simulink library "xblocks_library_pfbs"  (Simulink 7.6)
settings: Solver=ode45  SolverMode=SingleTasking  StartTime=0.0  StopTime=10.0  RelTol=1e-3
libraries: xbsIndex_r4 x369, monroe_library x47
(part 7 of 7)

== system xblocks_library_pfbs/pfb_fir/pfb_row_22/tap_split_2 ==
  inport : Inport
  Reinterp1 : xbsIndex_r4/Reinterpret  force_arith_type=on  arith_type="Signed  (2's comp)"  force_bin_pt=on  bin_pt=7  block_type=reinterpret
  Reinterp2 : xbsIndex_r4/Reinterpret  force_arith_type=on  arith_type="Signed  (2's comp)"  force_bin_pt=on  bin_pt=7  block_type=reinterpret
  Slice1 : xbsIndex_r4/Slice  nbits=8  boolean_output=off  mode=Upper Bit Location + Width  bit1=-0  base1=MSB of Input  bit0=0  base0=LSB of Input  dbl_ovrd=off  block_type=slice
  Slice2 : xbsIndex_r4/Slice  nbits=8  boolean_output=off  mode=Upper Bit Location + Width  bit1=-8  base1=MSB of Input  bit0=0  base0=LSB of Input  dbl_ovrd=off  block_type=slice
  outport1 : Outport
  outport2 : Outport  Port=2
  wires:
  inport/1 -> Slice2/1, Slice1/1
  Reinterp2/1 -> outport2/1
  Slice2/1 -> Reinterp2/1  "slice_out2"
  Reinterp1/1 -> outport1/1
  Slice1/1 -> Reinterp1/1  "slice_out1"

== system xblocks_library_pfbs/pfb_fir_real/coeff_gen_0_7/cram_lower ==
  in0 : Inport
  in1 : Inport  Port=2
  in2 : Inport  Port=3
  in3 : Inport  Port=4
  concat : xbsIndex_r4/Concat  num_inputs=4  dbl_ovrd=off  block_type=concat
  reinterpret_{1..4} (4 alike) : xbsIndex_r4/Reinterpret  force_arith_type=on  arith_type=Unsigned  force_bin_pt=on  bin_pt=0  block_type=reinterpret
  out : Outport
  wires:
  concat/1 -> out/1
  reinterpret_4/1 -> concat/4
  reinterpret_3/1 -> concat/3
  reinterpret_2/1 -> concat/2
  reinterpret_1/1 -> concat/1
  in3/1 -> reinterpret_4/1
  in2/1 -> reinterpret_3/1
  in1/1 -> reinterpret_2/1
  in0/1 -> reinterpret_1/1

== system xblocks_library_pfbs/pfb_fir_real/coeff_gen_0_7/cram_upper ==
  in0 : Inport
  in1 : Inport  Port=2
  in2 : Inport  Port=3
  in3 : Inport  Port=4
  concat : xbsIndex_r4/Concat  num_inputs=4  dbl_ovrd=off  block_type=concat
  reinterpret_{1..4} (4 alike) : xbsIndex_r4/Reinterpret  force_arith_type=on  arith_type=Unsigned  force_bin_pt=on  bin_pt=0  block_type=reinterpret
  out : Outport
  wires:
  concat/1 -> out/1
  reinterpret_4/1 -> concat/4
  reinterpret_3/1 -> concat/3
  reinterpret_2/1 -> concat/2
  reinterpret_1/1 -> concat/1
  in3/1 -> reinterpret_4/1
  in2/1 -> reinterpret_3/1
  in1/1 -> reinterpret_2/1
  in0/1 -> reinterpret_1/1

== system xblocks_library_pfbs/pfb_fir_real/coeff_gen_1_6/cram_lower ==
  in0 : Inport
  in1 : Inport  Port=2
  in2 : Inport  Port=3
  in3 : Inport  Port=4
  concat : xbsIndex_r4/Concat  num_inputs=4  dbl_ovrd=off  block_type=concat
  reinterpret_{1..4} (4 alike) : xbsIndex_r4/Reinterpret  force_arith_type=on  arith_type=Unsigned  force_bin_pt=on  bin_pt=0  block_type=reinterpret
  out : Outport
  wires:
  concat/1 -> out/1
  reinterpret_4/1 -> concat/4
  reinterpret_3/1 -> concat/3
  reinterpret_2/1 -> concat/2
  reinterpret_1/1 -> concat/1
  in3/1 -> reinterpret_4/1
  in2/1 -> reinterpret_3/1
  in1/1 -> reinterpret_2/1
  in0/1 -> reinterpret_1/1

== system xblocks_library_pfbs/pfb_fir_real/coeff_gen_1_6/cram_upper ==
  in0 : Inport
  in1 : Inport  Port=2
  in2 : Inport  Port=3
  in3 : Inport  Port=4
  concat : xbsIndex_r4/Concat  num_inputs=4  dbl_ovrd=off  block_type=concat
  reinterpret_{1..4} (4 alike) : xbsIndex_r4/Reinterpret  force_arith_type=on  arith_type=Unsigned  force_bin_pt=on  bin_pt=0  block_type=reinterpret
  out : Outport
  wires:
  concat/1 -> out/1
  reinterpret_4/1 -> concat/4
  reinterpret_3/1 -> concat/3
  reinterpret_2/1 -> concat/2
  reinterpret_1/1 -> concat/1
  in3/1 -> reinterpret_4/1
  in2/1 -> reinterpret_3/1
  in1/1 -> reinterpret_2/1
  in0/1 -> reinterpret_1/1

== system xblocks_library_pfbs/pfb_fir_real/coeff_gen_2_5/cram_lower ==
  in0 : Inport
  in1 : Inport  Port=2
  in2 : Inport  Port=3
  in3 : Inport  Port=4
  concat : xbsIndex_r4/Concat  num_inputs=4  dbl_ovrd=off  block_type=concat
  reinterpret_{1..4} (4 alike) : xbsIndex_r4/Reinterpret  force_arith_type=on  arith_type=Unsigned  force_bin_pt=on  bin_pt=0  block_type=reinterpret
  out : Outport
  wires:
  concat/1 -> out/1
  reinterpret_4/1 -> concat/4
  reinterpret_3/1 -> concat/3
  reinterpret_2/1 -> concat/2
  reinterpret_1/1 -> concat/1
  in3/1 -> reinterpret_4/1
  in2/1 -> reinterpret_3/1
  in1/1 -> reinterpret_2/1
  in0/1 -> reinterpret_1/1

== system xblocks_library_pfbs/pfb_fir_real/coeff_gen_2_5/cram_upper ==
  in0 : Inport
  in1 : Inport  Port=2
  in2 : Inport  Port=3
  in3 : Inport  Port=4
  concat : xbsIndex_r4/Concat  num_inputs=4  dbl_ovrd=off  block_type=concat
  reinterpret_{1..4} (4 alike) : xbsIndex_r4/Reinterpret  force_arith_type=on  arith_type=Unsigned  force_bin_pt=on  bin_pt=0  block_type=reinterpret
  out : Outport
  wires:
  concat/1 -> out/1
  reinterpret_4/1 -> concat/4
  reinterpret_3/1 -> concat/3
  reinterpret_2/1 -> concat/2
  reinterpret_1/1 -> concat/1
  in3/1 -> reinterpret_4/1
  in2/1 -> reinterpret_3/1
  in1/1 -> reinterpret_2/1
  in0/1 -> reinterpret_1/1

== system xblocks_library_pfbs/pfb_fir_real/coeff_gen_3_4/cram_lower ==
  in0 : Inport
  in1 : Inport  Port=2
  in2 : Inport  Port=3
  in3 : Inport  Port=4
  concat : xbsIndex_r4/Concat  num_inputs=4  dbl_ovrd=off  block_type=concat
  reinterpret_{1..4} (4 alike) : xbsIndex_r4/Reinterpret  force_arith_type=on  arith_type=Unsigned  force_bin_pt=on  bin_pt=0  block_type=reinterpret
  out : Outport
  wires:
  concat/1 -> out/1
  reinterpret_4/1 -> concat/4
  reinterpret_3/1 -> concat/3
  reinterpret_2/1 -> concat/2
  reinterpret_1/1 -> concat/1
  in3/1 -> reinterpret_4/1
  in2/1 -> reinterpret_3/1
  in1/1 -> reinterpret_2/1
  in0/1 -> reinterpret_1/1

== system xblocks_library_pfbs/pfb_fir_real/coeff_gen_3_4/cram_upper ==
  in0 : Inport
  in1 : Inport  Port=2
  in2 : Inport  Port=3
  in3 : Inport  Port=4
  concat : xbsIndex_r4/Concat  num_inputs=4  dbl_ovrd=off  block_type=concat
  reinterpret_{1..4} (4 alike) : xbsIndex_r4/Reinterpret  force_arith_type=on  arith_type=Unsigned  force_bin_pt=on  bin_pt=0  block_type=reinterpret
  out : Outport
  wires:
  concat/1 -> out/1
  reinterpret_4/1 -> concat/4
  reinterpret_3/1 -> concat/3
  reinterpret_2/1 -> concat/2
  reinterpret_1/1 -> concat/1
  in3/1 -> reinterpret_4/1
  in2/1 -> reinterpret_3/1
  in1/1 -> reinterpret_2/1
  in0/1 -> reinterpret_1/1

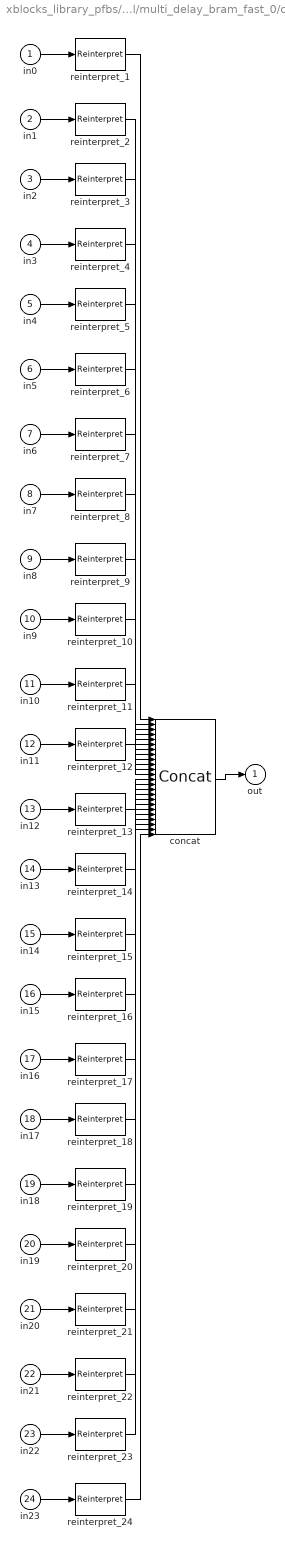
== system xblocks_library_pfbs/pfb_fir_real/multi_delay_bram_fast_0/cram ==
  in0 : Inport
  in1 : Inport  Port=2
  in2 : Inport  Port=3
  in3 : Inport  Port=4
  in4 : Inport  Port=5
  in5 : Inport  Port=6
  in6 : Inport  Port=7
  in7 : Inport  Port=8
  in8 : Inport  Port=9
  in9 : Inport  Port=10
  in10 : Inport  Port=11
  in11 : Inport  Port=12
  in12 : Inport  Port=13
  in13 : Inport  Port=14
  in14 : Inport  Port=15
  in15 : Inport  Port=16
  in16 : Inport  Port=17
  in17 : Inport  Port=18
  in18 : Inport  Port=19
  in19 : Inport  Port=20
  in20 : Inport  Port=21
  in21 : Inport  Port=22
  in22 : Inport  Port=23
  in23 : Inport  Port=24
  concat : xbsIndex_r4/Concat  num_inputs=24  dbl_ovrd=off  block_type=concat
  reinterpret_{1..24} (24 alike) : xbsIndex_r4/Reinterpret  force_arith_type=on  arith_type=Unsigned  force_bin_pt=on  bin_pt=0  block_type=reinterpret
  out : Outport
  wires:
  concat/1 -> out/1
  reinterpret_24/1 -> concat/24
  reinterpret_23/1 -> concat/23
  reinterpret_22/1 -> concat/22
  reinterpret_21/1 -> concat/21
  reinterpret_20/1 -> concat/20
  reinterpret_19/1 -> concat/19
  reinterpret_18/1 -> concat/18
  reinterpret_17/1 -> concat/17
  reinterpret_16/1 -> concat/16
  reinterpret_15/1 -> concat/15
  reinterpret_14/1 -> concat/14
  reinterpret_13/1 -> concat/13
  reinterpret_12/1 -> concat/12
  reinterpret_11/1 -> concat/11
  reinterpret_10/1 -> concat/10
  reinterpret_9/1 -> concat/9
  reinterpret_8/1 -> concat/8
  reinterpret_7/1 -> concat/7
  reinterpret_6/1 -> concat/6
  reinterpret_5/1 -> concat/5
  reinterpret_4/1 -> concat/4
  reinterpret_3/1 -> concat/3
  reinterpret_2/1 -> concat/2
  reinterpret_1/1 -> concat/1
  in23/1 -> reinterpret_24/1
  in22/1 -> reinterpret_23/1
  in21/1 -> reinterpret_22/1
  in20/1 -> reinterpret_21/1
  in19/1 -> reinterpret_20/1
  in18/1 -> reinterpret_19/1
  in17/1 -> reinterpret_18/1
  in16/1 -> reinterpret_17/1
  in15/1 -> reinterpret_16/1
  in14/1 -> reinterpret_15/1
  in13/1 -> reinterpret_14/1
  in12/1 -> reinterpret_13/1
  in11/1 -> reinterpret_12/1
  in10/1 -> reinterpret_11/1
  in9/1 -> reinterpret_10/1
  in8/1 -> reinterpret_9/1
  in7/1 -> reinterpret_8/1
  in6/1 -> reinterpret_7/1
  in5/1 -> reinterpret_6/1
  in4/1 -> reinterpret_5/1
  in3/1 -> reinterpret_4/1
  in2/1 -> reinterpret_3/1
  in1/1 -> reinterpret_2/1
  in0/1 -> reinterpret_1/1

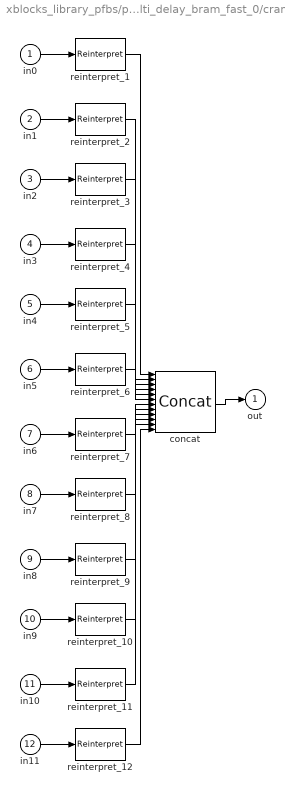
== system xblocks_library_pfbs/pfb_fir_real/multi_delay_bram_fast_0/cram_all ==
  in0 : Inport
  in1 : Inport  Port=2
  in2 : Inport  Port=3
  in3 : Inport  Port=4
  in4 : Inport  Port=5
  in5 : Inport  Port=6
  in6 : Inport  Port=7
  in7 : Inport  Port=8
  in8 : Inport  Port=9
  in9 : Inport  Port=10
  in10 : Inport  Port=11
  in11 : Inport  Port=12
  concat : xbsIndex_r4/Concat  num_inputs=12  dbl_ovrd=off  block_type=concat
  reinterpret_{1..12} (12 alike) : xbsIndex_r4/Reinterpret  force_arith_type=on  arith_type=Unsigned  force_bin_pt=on  bin_pt=0  block_type=reinterpret
  out : Outport
  wires:
  concat/1 -> out/1
  reinterpret_12/1 -> concat/12
  reinterpret_11/1 -> concat/11
  reinterpret_10/1 -> concat/10
  reinterpret_9/1 -> concat/9
  reinterpret_8/1 -> concat/8
  reinterpret_7/1 -> concat/7
  reinterpret_6/1 -> concat/6
  reinterpret_5/1 -> concat/5
  reinterpret_4/1 -> concat/4
  reinterpret_3/1 -> concat/3
  reinterpret_2/1 -> concat/2
  reinterpret_1/1 -> concat/1
  in11/1 -> reinterpret_12/1
  in10/1 -> reinterpret_11/1
  in9/1 -> reinterpret_10/1
  in8/1 -> reinterpret_9/1
  in7/1 -> reinterpret_8/1
  in6/1 -> reinterpret_7/1
  in5/1 -> reinterpret_6/1
  in4/1 -> reinterpret_5/1
  in3/1 -> reinterpret_4/1
  in2/1 -> reinterpret_3/1
  in1/1 -> reinterpret_2/1
  in0/1 -> reinterpret_1/1

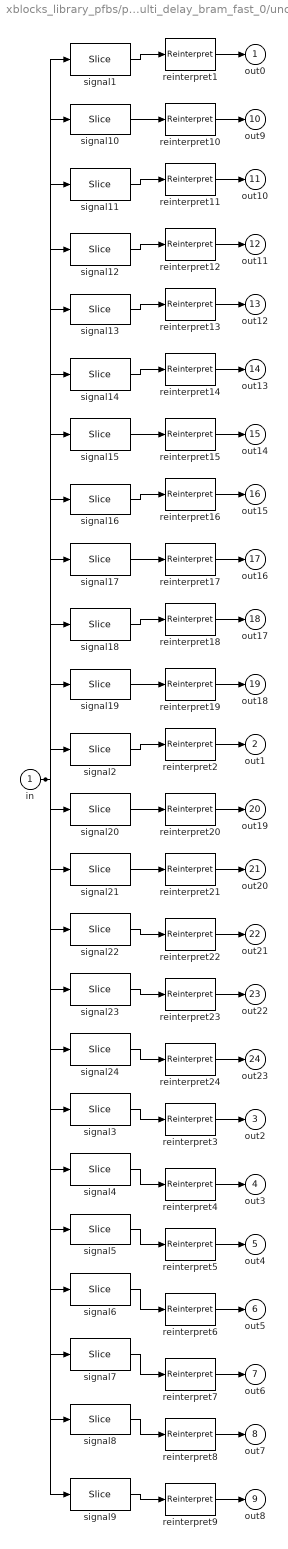
== system xblocks_library_pfbs/pfb_fir_real/multi_delay_bram_fast_0/uncram ==
  in : Inport
  reinterpret{1..24} (24 alike) : xbsIndex_r4/Reinterpret  force_arith_type=on  arith_type="Signed  (2's comp)"  force_bin_pt=on  bin_pt=17  block_type=reinterpret
  signal1 : xbsIndex_r4/Slice  nbits=18  boolean_output=off  mode=Upper Bit Location + Width  bit1=-0  base1=MSB of Input  bit0=-0  base0=MSB of Input  dbl_ovrd=off  block_type=slice
  signal10 : xbsIndex_r4/Slice  nbits=18  boolean_output=off  mode=Upper Bit Location + Width  bit1=-162  base1=MSB of Input  bit0=-162  base0=MSB of Input  dbl_ovrd=off  block_type=slice
  signal11 : xbsIndex_r4/Slice  nbits=18  boolean_output=off  mode=Upper Bit Location + Width  bit1=-180  base1=MSB of Input  bit0=-180  base0=MSB of Input  dbl_ovrd=off  block_type=slice
  signal12 : xbsIndex_r4/Slice  nbits=18  boolean_output=off  mode=Upper Bit Location + Width  bit1=-198  base1=MSB of Input  bit0=-198  base0=MSB of Input  dbl_ovrd=off  block_type=slice
  signal13 : xbsIndex_r4/Slice  nbits=18  boolean_output=off  mode=Upper Bit Location + Width  bit1=-216  base1=MSB of Input  bit0=-216  base0=MSB of Input  dbl_ovrd=off  block_type=slice
  signal14 : xbsIndex_r4/Slice  nbits=18  boolean_output=off  mode=Upper Bit Location + Width  bit1=-234  base1=MSB of Input  bit0=-234  base0=MSB of Input  dbl_ovrd=off  block_type=slice
  signal15 : xbsIndex_r4/Slice  nbits=18  boolean_output=off  mode=Upper Bit Location + Width  bit1=-252  base1=MSB of Input  bit0=-252  base0=MSB of Input  dbl_ovrd=off  block_type=slice
  signal16 : xbsIndex_r4/Slice  nbits=18  boolean_output=off  mode=Upper Bit Location + Width  bit1=-270  base1=MSB of Input  bit0=-270  base0=MSB of Input  dbl_ovrd=off  block_type=slice
  signal17 : xbsIndex_r4/Slice  nbits=18  boolean_output=off  mode=Upper Bit Location + Width  bit1=-288  base1=MSB of Input  bit0=-288  base0=MSB of Input  dbl_ovrd=off  block_type=slice
  signal18 : xbsIndex_r4/Slice  nbits=18  boolean_output=off  mode=Upper Bit Location + Width  bit1=-306  base1=MSB of Input  bit0=-306  base0=MSB of Input  dbl_ovrd=off  block_type=slice
  signal19 : xbsIndex_r4/Slice  nbits=18  boolean_output=off  mode=Upper Bit Location + Width  bit1=-324  base1=MSB of Input  bit0=-324  base0=MSB of Input  dbl_ovrd=off  block_type=slice
  signal2 : xbsIndex_r4/Slice  nbits=18  boolean_output=off  mode=Upper Bit Location + Width  bit1=-18  base1=MSB of Input  bit0=-18  base0=MSB of Input  dbl_ovrd=off  block_type=slice
  signal20 : xbsIndex_r4/Slice  nbits=18  boolean_output=off  mode=Upper Bit Location + Width  bit1=-342  base1=MSB of Input  bit0=-342  base0=MSB of Input  dbl_ovrd=off  block_type=slice
  signal21 : xbsIndex_r4/Slice  nbits=18  boolean_output=off  mode=Upper Bit Location + Width  bit1=-360  base1=MSB of Input  bit0=-360  base0=MSB of Input  dbl_ovrd=off  block_type=slice
  signal22 : xbsIndex_r4/Slice  nbits=18  boolean_output=off  mode=Upper Bit Location + Width  bit1=-378  base1=MSB of Input  bit0=-378  base0=MSB of Input  dbl_ovrd=off  block_type=slice
  signal23 : xbsIndex_r4/Slice  nbits=18  boolean_output=off  mode=Upper Bit Location + Width  bit1=-396  base1=MSB of Input  bit0=-396  base0=MSB of Input  dbl_ovrd=off  block_type=slice
  signal24 : xbsIndex_r4/Slice  nbits=18  boolean_output=off  mode=Upper Bit Location + Width  bit1=-414  base1=MSB of Input  bit0=-414  base0=MSB of Input  dbl_ovrd=off  block_type=slice
  signal3 : xbsIndex_r4/Slice  nbits=18  boolean_output=off  mode=Upper Bit Location + Width  bit1=-36  base1=MSB of Input  bit0=-36  base0=MSB of Input  dbl_ovrd=off  block_type=slice
  signal4 : xbsIndex_r4/Slice  nbits=18  boolean_output=off  mode=Upper Bit Location + Width  bit1=-54  base1=MSB of Input  bit0=-54  base0=MSB of Input  dbl_ovrd=off  block_type=slice
  signal5 : xbsIndex_r4/Slice  nbits=18  boolean_output=off  mode=Upper Bit Location + Width  bit1=-72  base1=MSB of Input  bit0=-72  base0=MSB of Input  dbl_ovrd=off  block_type=slice
  signal6 : xbsIndex_r4/Slice  nbits=18  boolean_output=off  mode=Upper Bit Location + Width  bit1=-90  base1=MSB of Input  bit0=-90  base0=MSB of Input  dbl_ovrd=off  block_type=slice
  signal7 : xbsIndex_r4/Slice  nbits=18  boolean_output=off  mode=Upper Bit Location + Width  bit1=-108  base1=MSB of Input  bit0=-108  base0=MSB of Input  dbl_ovrd=off  block_type=slice
  signal8 : xbsIndex_r4/Slice  nbits=18  boolean_output=off  mode=Upper Bit Location + Width  bit1=-126  base1=MSB of Input  bit0=-126  base0=MSB of Input  dbl_ovrd=off  block_type=slice
  signal9 : xbsIndex_r4/Slice  nbits=18  boolean_output=off  mode=Upper Bit Location + Width  bit1=-144  base1=MSB of Input  bit0=-144  base0=MSB of Input  dbl_ovrd=off  block_type=slice
  out0 : Outport
  out1 : Outport  Port=2
  out2 : Outport  Port=3
  out3 : Outport  Port=4
  out4 : Outport  Port=5
  out5 : Outport  Port=6
  out6 : Outport  Port=7
  out7 : Outport  Port=8
  out8 : Outport  Port=9
  out9 : Outport  Port=10
  out10 : Outport  Port=11
  out11 : Outport  Port=12
  out12 : Outport  Port=13
  out13 : Outport  Port=14
  out14 : Outport  Port=15
  out15 : Outport  Port=16
  out16 : Outport  Port=17
  out17 : Outport  Port=18
  out18 : Outport  Port=19
  out19 : Outport  Port=20
  out20 : Outport  Port=21
  out21 : Outport  Port=22
  out22 : Outport  Port=23
  out23 : Outport  Port=24
  wires:
  in/1 -> signal24/1, signal23/1, signal22/1, signal21/1, signal20/1, signal19/1, signal18/1, signal17/1, signal16/1, signal15/1, signal14/1, signal13/1, signal12/1, signal11/1, signal10/1, signal9/1, signal8/1, signal7/1, signal6/1, signal5/1, signal4/1, signal3/1, signal2/1, signal1/1
  reinterpret24/1 -> out23/1
  signal24/1 -> reinterpret24/1
  reinterpret23/1 -> out22/1
  signal23/1 -> reinterpret23/1
  reinterpret22/1 -> out21/1
  signal22/1 -> reinterpret22/1
  reinterpret21/1 -> out20/1
  signal21/1 -> reinterpret21/1
  reinterpret20/1 -> out19/1
  signal20/1 -> reinterpret20/1
  reinterpret19/1 -> out18/1
  signal19/1 -> reinterpret19/1
  reinterpret18/1 -> out17/1
  signal18/1 -> reinterpret18/1
  reinterpret17/1 -> out16/1
  signal17/1 -> reinterpret17/1
  reinterpret16/1 -> out15/1
  signal16/1 -> reinterpret16/1
  reinterpret15/1 -> out14/1
  signal15/1 -> reinterpret15/1
  reinterpret14/1 -> out13/1
  signal14/1 -> reinterpret14/1
  reinterpret13/1 -> out12/1
  signal13/1 -> reinterpret13/1
  reinterpret12/1 -> out11/1
  signal12/1 -> reinterpret12/1
  reinterpret11/1 -> out10/1
  signal11/1 -> reinterpret11/1
  reinterpret10/1 -> out9/1
  signal10/1 -> reinterpret10/1
  reinterpret9/1 -> out8/1
  signal9/1 -> reinterpret9/1
  reinterpret8/1 -> out7/1
  signal8/1 -> reinterpret8/1
  reinterpret7/1 -> out6/1
  signal7/1 -> reinterpret7/1
  reinterpret6/1 -> out5/1
  signal6/1 -> reinterpret6/1
  reinterpret5/1 -> out4/1
  signal5/1 -> reinterpret5/1
  reinterpret4/1 -> out3/1
  signal4/1 -> reinterpret4/1
  reinterpret3/1 -> out2/1
  signal3/1 -> reinterpret3/1
  reinterpret2/1 -> out1/1
  signal2/1 -> reinterpret2/1
  reinterpret1/1 -> out0/1
  signal1/1 -> reinterpret1/1
